simulink model "TorqueVect"  (R2022a)
settings: Solver=VariableStepAuto  StartTime=0.0  StopTime=32  RelTol=1e-3
PreLoadFcn:
  | run('Parameters\FSE_Parameters.m')
undefined symbols (not defined in the file): BRegenEnabledButton, canChannel, CyalphaLookUp, efficiency, Fz_curve, Fz_scaling_long, gearR, izz, jw, Kd, kd, Ki, ki, Kp, kp, l_f, l_r, lambda, m, Mz_max, N, N_lat, N_long, P_max, pid_kd_lat, pid_kd_long, pid_ki_lat, pid_ki_long, pid_kp_lat, pid_kp_long, R_max, rw, steerR, T_i_max, TC_Decr_Gas, TC_Derivative, TC_Incr_Gas, TC_On, TC_Relay_Off, TC_Relay_On, tireCornerStiffness, Ts, TV_On, TV_Override, velocity_lookup, velocity_lookup_lat, y_ref, yrr_scaling
libraries: simulink x218, slpidlib x135, CarMaker4SL x101, TractionControlLibrary x13, canmsglib x9, canlib x8, TorqueVectoringLibrary x6, simulink_extras x4, PedalConversionLibrary x3, PowerControlLibrary x1
(part 6 of 26)

== system TorqueVect/CarMaker/IPG Vehicle/PowerTrain/PTControl Example/PTControl_PC_MFE/New TC ==
  lim 1 : Inport
  lim 2 : Inport  Port=2
  lim 3 : Inport  Port=3
  lim 4 : Inport  Port=4
  vx : Inport  Port=5
  w_FL : Inport  Port=6
  w_FR : Inport  Port=7
  w_RL : Inport  Port=8
  w_RR : Inport  Port=9
  Front SR Target : Inport  Port=10
  Rear SR Target : Inport  Port=11
  P_TC : Inport  Port=12
  D_TC : Inport  Port=13
  enable_tc : Inport  Port=14
  rate_h : Inport  Port=15
  rate_l : Inport  Port=16
  Demux1 : Demux
  Gain : Gain  Gain=0.2032/13.39
  Rate Limiter Dynamic{,1..3} (4 alike) : simulink/Discontinuities/Rate Limiter Dynamic
  Reference Generator1 : Subsystem
  Saturation : Saturate  UpperLimit=inf  LowerLimit=0
  Subtract1 : Sum  Inputs=-+
  TC R1 : Subsystem
  TC R2 : Subsystem
  TC R3 : Subsystem
  TC R4 : Subsystem
  Vector Concatenate3 : Concatenate  NumInputs=4
  R1 Demand : Outport
  L1 Demand : Outport  Port=2
  R2 Demand : Outport  Port=3
  L2 Demand : Outport  Port=4
  wires:
  Reference Generator1/1(R1) -> TC R1/1(modified slip ratio reference)
  lim 1/1 -> TC R1/2(lim 1)
  Gain/1 -> Subtract1/2
  Vector Concatenate3/1 -> Gain/1  "omega"
  Subtract1/1 -> Demux1/1
  vx/1 -> Saturation/1
  TC R2/1(Control Effort 1) -> Rate Limiter Dynamic1/2  "MMotorL1Demand"
  w_RL/1 -> Vector Concatenate3/4
  w_RR/1 -> Vector Concatenate3/3
  w_FL/1 -> Vector Concatenate3/2
  w_FR/1 -> Vector Concatenate3/1
  Front SR Target/1 -> Reference Generator1/2(Front SR Target)
  Rear SR Target/1 -> Reference Generator1/3(Rear SR Target)
  lim 2/1 -> TC R2/2(lim 1)
  lim 3/1 -> TC R3/2(lim 1)
  lim 4/1 -> TC R4/2(lim 1)
  Reference Generator1/2(L1) -> TC R2/1(modified slip ratio reference)
  Reference Generator1/3(R2) -> TC R3/1(modified slip ratio reference)
  Reference Generator1/4(L2) -> TC R4/1(modified slip ratio reference)
  P_TC/1 -> TC R2/4(P_TC), TC R4/4(P_TC), TC R3/4(P_TC), TC R1/4(P_TC)
  D_TC/1 -> TC R2/5(D_TC), TC R4/5(D_TC), TC R3/5(D_TC), TC R1/5(D_TC)
  Demux1/1 -> TC R1/3(modified slip ratio measurement)
  Demux1/2 -> TC R2/3(modified slip ratio measurement)
  Demux1/3 -> TC R3/3(modified slip ratio measurement)
  Demux1/4 -> TC R4/3(modified slip ratio measurement)
  TC R1/1(Control Effort 1) -> Rate Limiter Dynamic/2  "MMotorR1Demand"
  Saturation/1 -> Subtract1/1, Reference Generator1/1(x2)
  TC R3/1(Control Effort 1) -> Rate Limiter Dynamic2/2
  TC R4/1(Control Effort 1) -> Rate Limiter Dynamic3/2
  enable_tc/1 -> TC R4/6(enable_tc), TC R2/6(enable_tc), TC R3/6(enable_tc), TC R1/6(enable_tc)
  Rate Limiter Dynamic/1 -> R1 Demand/1
  rate_h/1 -> Rate Limiter Dynamic3/1, Rate Limiter Dynamic2/1, Rate Limiter Dynamic1/1, Rate Limiter Dynamic/1
  rate_l/1 -> Rate Limiter Dynamic/3, Rate Limiter Dynamic3/3, Rate Limiter Dynamic2/3, Rate Limiter Dynamic1/3
  Rate Limiter Dynamic1/1 -> L1 Demand/1
  Rate Limiter Dynamic2/1 -> R2 Demand/1
  Rate Limiter Dynamic3/1 -> L2 Demand/1

== system TorqueVect/CarMaker/IPG Vehicle/PowerTrain/PTControl Example/PTControl_PC_MFE/PTC ==
  Constant2 : Constant
  Ground : Ground
  Mode_EngineDrive : Constant  Value=4
  Mux : Mux
  OperState_Driving : Constant  Value=4
  PTC MiscOut : Outport  VectorParamsAs1DForOutWhenUnconnected=off
  wires:
  Constant2/1 -> Mux/4  "Ignition"
  Mode_EngineDrive/1 -> Mux/3
  Ground/1 -> Mux/2  "OperationError"
  OperState_Driving/1 -> Mux/1
  Mux/1 -> PTC MiscOut/1

== system TorqueVect/CarMaker/IPG Vehicle/PowerTrain/PTControl Example/PTControl_PC_MFE/Subsystem ==
  rThrottlePedal : Inport
  vLong : Inport  Port=2
  BRegenEnabledButton : Inport  Port=3
  MMotorFL : Inport  Port=4
  MMotorFR : Inport  Port=5
  MMotorRL : Inport  Port=6
  MMotorRR : Inport  Port=7
  nMotorFL : Inport  Port=8
  nMotorFR : Inport  Port=9
  nMotorRL : Inport  Port=10
  nMotorRR : Inport  Port=11
  PMeasured : Inport  Port=12
  BMeasuredEnable : Inport  Port=13
  rSplitF : Inport  Port=14
  rRegenSplitF : Inport  Port=15
  PRegenLimit : Inport  Port=16
  PLimit : Inport  Port=17
  FF_PC : Inport  Port=18
  FF_RC : Inport  Port=19
  P_PC : Inport  Port=20
  D_PC : Inport  Port=21
  MMotorMax : Inport  Port=22
  Add{,1..3} (4 alike) : Sum  Inputs=-+
  PedalConversion : PedalConversionLibrary/PedalConversion  SystemSampleTime=-1  VariantActivationTime=update diagram  Latency=0  AutoFrameSizeCalculation=off
  PowerControl : Subsystem  AncestorBlock=PowerControlLibrary/PowerControl
  TorqueSplit : TorqueVectoringLibrary/TorqueSplit  SystemSampleTime=-1  VariantActivationTime=update diagram  Latency=0  AutoFrameSizeCalculation=off
  MMotorDemandFL : Outport
  MMotorDemandFR : Outport  Port=2
  MMotorDemandRL : Outport  Port=3
  MMotorDemandRR : Outport  Port=4
  wires:
  rThrottlePedal/1 -> [rThrottlePedal]
  [rThrottlePedal] -> PedalConversion/1
  [rThrottlePedal] -> PowerControl/13(rThrottlePedal)
  vLong/1 -> PedalConversion/3
  BRegenEnabledButton/1 -> PedalConversion/2
  MMotorFL/1 -> PowerControl/1(MMotorFL)
  MMotorFR/1 -> PowerControl/2(MMotorFR)
  MMotorRL/1 -> PowerControl/3(MMotorRL)
  MMotorRR/1 -> PowerControl/4(MMotorRR)
  nMotorFL/1 -> PowerControl/5(nMotorFL)
  nMotorFR/1 -> PowerControl/6(nMotorFR)
  nMotorRL/1 -> PowerControl/7(nMotorRL)
  nMotorRR/1 -> PowerControl/8(nMotorRR)
  PMeasured/1 -> PowerControl/9(PMeasured)
  BMeasuredEnable/1 -> PowerControl/10(BMeasuredEnable)
  PRegenLimit/1 -> PowerControl/15(PRegenLimit)
  PLimit/1 -> PowerControl/16(PLimit)
  FF_PC/1 -> PowerControl/17(FF_PC)
  FF_RC/1 -> PowerControl/18(FF_RC)
  P_PC/1 -> PowerControl/19(P_PC)
  D_PC/1 -> PowerControl/20(D_PC)
  Add/1 -> MMotorDemandFL/1
  PowerControl/1(MReductionMotorFL) -> Add/1
  rSplitF/1 -> [rSplitF]
  [rSplitF] -> TorqueSplit/1
  rRegenSplitF/1 -> TorqueSplit/2
  PedalConversion/1 -> PowerControl/14(rThrottle), TorqueSplit/3
  MMotorMax/1 -> TorqueSplit/4
  [rSplitF] -> PowerControl/12(rSplitF)
  PedalConversion/2 -> PowerControl/11(BRegenEnable)
  TorqueSplit/1 -> [MMotorRequestFL]
  TorqueSplit/2 -> [MMotorRequestFR]
  TorqueSplit/3 -> [MMotorRequestRL]
  TorqueSplit/4 -> [MMotorRequestRR]
  [MMotorRequestFL] -> Add/2
  Add1/1 -> MMotorDemandFR/1
  PowerControl/2(MReductionMotorFR) -> Add1/1
  [MMotorRequestFR] -> Add1/2
  Add2/1 -> MMotorDemandRL/1
  PowerControl/3(MReductionMotorRL) -> Add2/1
  [MMotorRequestRL] -> Add2/2
  Add3/1 -> MMotorDemandRR/1
  PowerControl/4(MReductionMotorRR) -> Add3/1
  [MMotorRequestRR] -> Add3/2

== system TorqueVect/CarMaker/IPG Vehicle/PowerTrain/PTControl Example/PTControl_PC_TC_MFE/New TC ==
  lim 1 : Inport
  lim 2 : Inport  Port=2
  lim 3 : Inport  Port=3
  lim 4 : Inport  Port=4
  vx : Inport  Port=5
  w_FL : Inport  Port=6
  w_FR : Inport  Port=7
  w_RL : Inport  Port=8
  w_RR : Inport  Port=9
  Front SR Target : Inport  Port=10
  Rear SR Target : Inport  Port=11
  P_TC : Inport  Port=12
  D_TC : Inport  Port=13
  enable_tc : Inport  Port=14
  rate_h : Inport  Port=15
  rate_l : Inport  Port=16
  Demux1 : Demux
  Gain : Gain  Gain=0.2032/13.39
  Rate Limiter Dynamic{,1..3} (4 alike) : simulink/Discontinuities/Rate Limiter Dynamic
  Reference Generator1 : Subsystem
  Saturation : Saturate  UpperLimit=inf  LowerLimit=0
  Subtract1 : Sum  Inputs=-+
  TC R1 : Subsystem
  TC R2 : Subsystem
  TC R3 : Subsystem
  TC R4 : Subsystem
  Vector Concatenate3 : Concatenate  NumInputs=4
  R1 Demand : Outport
  L1 Demand : Outport  Port=2
  R2 Demand : Outport  Port=3
  L2 Demand : Outport  Port=4
  wires:
  Reference Generator1/1(R1) -> TC R1/1(modified slip ratio reference)
  lim 1/1 -> TC R1/2(lim 1)
  Gain/1 -> Subtract1/2
  Vector Concatenate3/1 -> Gain/1  "omega"
  Subtract1/1 -> Demux1/1
  vx/1 -> Saturation/1
  TC R2/1(Control Effort 1) -> Rate Limiter Dynamic1/2  "MMotorL1Demand"
  w_RL/1 -> Vector Concatenate3/4
  w_RR/1 -> Vector Concatenate3/3
  w_FL/1 -> Vector Concatenate3/2
  w_FR/1 -> Vector Concatenate3/1
  Front SR Target/1 -> Reference Generator1/2(Front SR Target)
  Rear SR Target/1 -> Reference Generator1/3(Rear SR Target)
  lim 2/1 -> TC R2/2(lim 1)
  lim 3/1 -> TC R3/2(lim 1)
  lim 4/1 -> TC R4/2(lim 1)
  Reference Generator1/2(L1) -> TC R2/1(modified slip ratio reference)
  Reference Generator1/3(R2) -> TC R3/1(modified slip ratio reference)
  Reference Generator1/4(L2) -> TC R4/1(modified slip ratio reference)
  P_TC/1 -> TC R2/4(P_TC), TC R4/4(P_TC), TC R3/4(P_TC), TC R1/4(P_TC)
  D_TC/1 -> TC R2/5(D_TC), TC R4/5(D_TC), TC R3/5(D_TC), TC R1/5(D_TC)
  Demux1/1 -> TC R1/3(modified slip ratio measurement)
  Demux1/2 -> TC R2/3(modified slip ratio measurement)
  Demux1/3 -> TC R3/3(modified slip ratio measurement)
  Demux1/4 -> TC R4/3(modified slip ratio measurement)
  TC R1/1(Control Effort 1) -> Rate Limiter Dynamic/2  "MMotorR1Demand"
  Saturation/1 -> Subtract1/1, Reference Generator1/1(x2)
  TC R3/1(Control Effort 1) -> Rate Limiter Dynamic2/2
  TC R4/1(Control Effort 1) -> Rate Limiter Dynamic3/2
  enable_tc/1 -> TC R4/6(enable_tc), TC R2/6(enable_tc), TC R3/6(enable_tc), TC R1/6(enable_tc)
  Rate Limiter Dynamic/1 -> R1 Demand/1
  rate_h/1 -> Rate Limiter Dynamic3/1, Rate Limiter Dynamic2/1, Rate Limiter Dynamic1/1, Rate Limiter Dynamic/1
  rate_l/1 -> Rate Limiter Dynamic/3, Rate Limiter Dynamic3/3, Rate Limiter Dynamic2/3, Rate Limiter Dynamic1/3
  Rate Limiter Dynamic1/1 -> L1 Demand/1
  Rate Limiter Dynamic2/1 -> R2 Demand/1
  Rate Limiter Dynamic3/1 -> L2 Demand/1

== system TorqueVect/CarMaker/IPG Vehicle/PowerTrain/PTControl Example/PTControl_PC_TC_MFE/PTC ==
  Constant2 : Constant
  Ground : Ground
  Mode_EngineDrive : Constant  Value=4
  Mux : Mux
  OperState_Driving : Constant  Value=4
  PTC MiscOut : Outport  VectorParamsAs1DForOutWhenUnconnected=off
  wires:
  Constant2/1 -> Mux/4  "Ignition"
  Mode_EngineDrive/1 -> Mux/3
  Ground/1 -> Mux/2  "OperationError"
  OperState_Driving/1 -> Mux/1
  Mux/1 -> PTC MiscOut/1

== system TorqueVect/CarMaker/IPG Vehicle/PowerTrain/PTControl Example/PTControl_PC_TC_MFE/Subsystem1 ==
  rThrottlePedal : Inport
  vLong : Inport  Port=2
  BRegenEnabledButton : Inport  Port=3
  MMotorFL : Inport  Port=4
  MMotorFR : Inport  Port=5
  MMotorRL : Inport  Port=6
  MMotorRR : Inport  Port=7
  rSlipTargetF : Inport  Port=8
  rSlipTargetR : Inport  Port=9
  BEnableTC : Inport  Port=10
  P_TC : Inport  Port=11
  PMeasured : Inport  Port=12
  D_TC : Inport  Port=13
  BMeasuredEnable : Inport  Port=14
  FF_TC : Inport  Port=15
  rSplitF : Inport  Port=16
  rLimitHigh : Inport  Port=17
  rRegenSplitF : Inport  Port=18
  PRegenLimit : Inport  Port=19
  rLimitLow : Inport  Port=20
  PLimit : Inport  Port=21
  FF_PC : Inport  Port=22
  FF_RC : Inport  Port=23
  P_PC : Inport  Port=24
  D_PC : Inport  Port=25
  MMotorMax : Inport  Port=26
  nMotorFL : Inport  Port=27
  nMotorFR : Inport  Port=28
  nMotorRL : Inport  Port=29
  nMotorRR : Inport  Port=30
  Subsystem : Subsystem
  TC : Subsystem
  MMotorDemandFL : Outport
  MMotorDemandFR : Outport  Port=2
  MMotorDemandRL : Outport  Port=3
  MMotorDemandRR : Outport  Port=4
  wires:
  [nMotorRL] -> Subsystem/10(nMotorRL)
  PRegenLimit/1 -> Subsystem/16(PRegenLimit)
  Subsystem/1(MMotorDemandFL) -> TC/14(MMotorRequestFL)
  [nMotorFL] -> Subsystem/8(nMotorFL)
  FF_TC/1 -> TC/11(FF_TC)
  Subsystem/3(MMotorDemandRL) -> TC/16(MMotorRequestRL)
  Subsystem/2(MMotorDemandFR) -> TC/15(MMotorRequestFR)
  rRegenSplitF/1 -> Subsystem/15(rRegenSplitF)
  BMeasuredEnable/1 -> Subsystem/13(BMeasuredEnable)
  MMotorMax/1 -> Subsystem/22(MMotorMax)
  Subsystem/4(MMotorDemandRR) -> TC/17(MMotorRequestRR)
  FF_PC/1 -> Subsystem/18(FF_PC)
  D_PC/1 -> Subsystem/21(D_PC)
  rLimitLow/1 -> TC/13(rLimitLow)
  TC/3(MMotorDemandRL) -> MMotorDemandRL/1
  [nMotorFR] -> Subsystem/9(nMotorFR)
  TC/4(MMotorDemandRR) -> MMotorDemandRR/1
  D_TC/1 -> TC/10(D_TC)
  PLimit/1 -> Subsystem/17(PLimit)
  P_PC/1 -> Subsystem/20(P_PC)
  FF_RC/1 -> Subsystem/19(FF_RC)
  vLong/1 -> TC/1(vLong), Subsystem/2(vLong)
  [nMotorFL] -> TC/2(nMotorFL)
  [nMotorRL] -> TC/4(nMotorRL)
  TC/1(MMotorDemandFL) -> MMotorDemandFL/1
  MMotorRL/1 -> Subsystem/6(MMotorRL)
  P_TC/1 -> TC/9(P_TC)
  MMotorFL/1 -> Subsystem/4(MMotorFL)
  [nMotorFR] -> TC/3(nMotorFR)
  [nMotorRR] -> TC/5(nMotorRR)
  rSlipTargetF/1 -> TC/6(rSlipTargetF)
  rSlipTargetR/1 -> TC/7(rSlipTargetR)
  rLimitHigh/1 -> TC/12(rLimitHigh)
  BEnableTC/1 -> TC/8(BEnableTC)
  BRegenEnabledButton/1 -> Subsystem/3(BRegenEnabledButton)
  rSplitF/1 -> Subsystem/14(rSplitF)
  [nMotorRR] -> Subsystem/11(nMotorRR)
  MMotorFR/1 -> Subsystem/5(MMotorFR)
  MMotorRR/1 -> Subsystem/7(MMotorRR)
  TC/2(MMotorDemandFR) -> MMotorDemandFR/1
  rThrottlePedal/1 -> Subsystem/1(rThrottlePedal)
  PMeasured/1 -> Subsystem/12(PMeasured)
  nMotorFL/1 -> [nMotorFL]
  nMotorFR/1 -> [nMotorFR]
  nMotorRL/1 -> [nMotorRL]
  nMotorRR/1 -> [nMotorRR]

== system TorqueVect/CarMaker/IPG Vehicle/PowerTrain/PTControl Example/PTControl_TC_MFE/New TC ==
  lim 1 : Inport
  lim 2 : Inport  Port=2
  lim 3 : Inport  Port=3
  lim 4 : Inport  Port=4
  vx : Inport  Port=5
  w_FL : Inport  Port=6
  w_FR : Inport  Port=7
  w_RL : Inport  Port=8
  w_RR : Inport  Port=9
  Front SR Target : Inport  Port=10
  Rear SR Target : Inport  Port=11
  P_TC : Inport  Port=12
  D_TC : Inport  Port=13
  enable_tc : Inport  Port=14
  rate_h : Inport  Port=15
  rate_l : Inport  Port=16
  Demux1 : Demux
  Gain : Gain  Gain=0.2032/13.39
  Rate Limiter Dynamic{,1..3} (4 alike) : simulink/Discontinuities/Rate Limiter Dynamic
  Reference Generator1 : Subsystem
  Saturation : Saturate  UpperLimit=inf  LowerLimit=0
  Subtract1 : Sum  Inputs=-+
  TC R1 : Subsystem
  TC R2 : Subsystem
  TC R3 : Subsystem
  TC R4 : Subsystem
  Vector Concatenate3 : Concatenate  NumInputs=4
  R1 Demand : Outport
  L1 Demand : Outport  Port=2
  R2 Demand : Outport  Port=3
  L2 Demand : Outport  Port=4
  wires:
  Reference Generator1/1(R1) -> TC R1/1(modified slip ratio reference)
  lim 1/1 -> TC R1/2(lim 1)
  Gain/1 -> Subtract1/2
  Vector Concatenate3/1 -> Gain/1  "omega"
  Subtract1/1 -> Demux1/1
  vx/1 -> Saturation/1
  TC R2/1(Control Effort 1) -> Rate Limiter Dynamic1/2  "MMotorL1Demand"
  w_RL/1 -> Vector Concatenate3/4
  w_RR/1 -> Vector Concatenate3/3
  w_FL/1 -> Vector Concatenate3/2
  w_FR/1 -> Vector Concatenate3/1
  Front SR Target/1 -> Reference Generator1/2(Front SR Target)
  Rear SR Target/1 -> Reference Generator1/3(Rear SR Target)
  lim 2/1 -> TC R2/2(lim 1)
  lim 3/1 -> TC R3/2(lim 1)
  lim 4/1 -> TC R4/2(lim 1)
  Reference Generator1/2(L1) -> TC R2/1(modified slip ratio reference)
  Reference Generator1/3(R2) -> TC R3/1(modified slip ratio reference)
  Reference Generator1/4(L2) -> TC R4/1(modified slip ratio reference)
  P_TC/1 -> TC R2/4(P_TC), TC R4/4(P_TC), TC R3/4(P_TC), TC R1/4(P_TC)
  D_TC/1 -> TC R2/5(D_TC), TC R4/5(D_TC), TC R3/5(D_TC), TC R1/5(D_TC)
  Demux1/1 -> TC R1/3(modified slip ratio measurement)
  Demux1/2 -> TC R2/3(modified slip ratio measurement)
  Demux1/3 -> TC R3/3(modified slip ratio measurement)
  Demux1/4 -> TC R4/3(modified slip ratio measurement)
  TC R1/1(Control Effort 1) -> Rate Limiter Dynamic/2  "MMotorR1Demand"
  Saturation/1 -> Subtract1/1, Reference Generator1/1(x2)
  TC R3/1(Control Effort 1) -> Rate Limiter Dynamic2/2
  TC R4/1(Control Effort 1) -> Rate Limiter Dynamic3/2
  enable_tc/1 -> TC R4/6(enable_tc), TC R2/6(enable_tc), TC R3/6(enable_tc), TC R1/6(enable_tc)
  Rate Limiter Dynamic/1 -> R1 Demand/1
  rate_h/1 -> Rate Limiter Dynamic3/1, Rate Limiter Dynamic2/1, Rate Limiter Dynamic1/1, Rate Limiter Dynamic/1
  rate_l/1 -> Rate Limiter Dynamic/3, Rate Limiter Dynamic3/3, Rate Limiter Dynamic2/3, Rate Limiter Dynamic1/3
  Rate Limiter Dynamic1/1 -> L1 Demand/1
  Rate Limiter Dynamic2/1 -> R2 Demand/1
  Rate Limiter Dynamic3/1 -> L2 Demand/1

== system TorqueVect/CarMaker/IPG Vehicle/PowerTrain/PTControl Example/PTControl_TC_MFE/PTC ==
  Constant2 : Constant
  Ground : Ground
  Mode_EngineDrive : Constant  Value=4
  Mux : Mux
  OperState_Driving : Constant  Value=4
  PTC MiscOut : Outport  VectorParamsAs1DForOutWhenUnconnected=off
  wires:
  Constant2/1 -> Mux/4  "Ignition"
  Mode_EngineDrive/1 -> Mux/3
  Ground/1 -> Mux/2  "OperationError"
  OperState_Driving/1 -> Mux/1
  Mux/1 -> PTC MiscOut/1

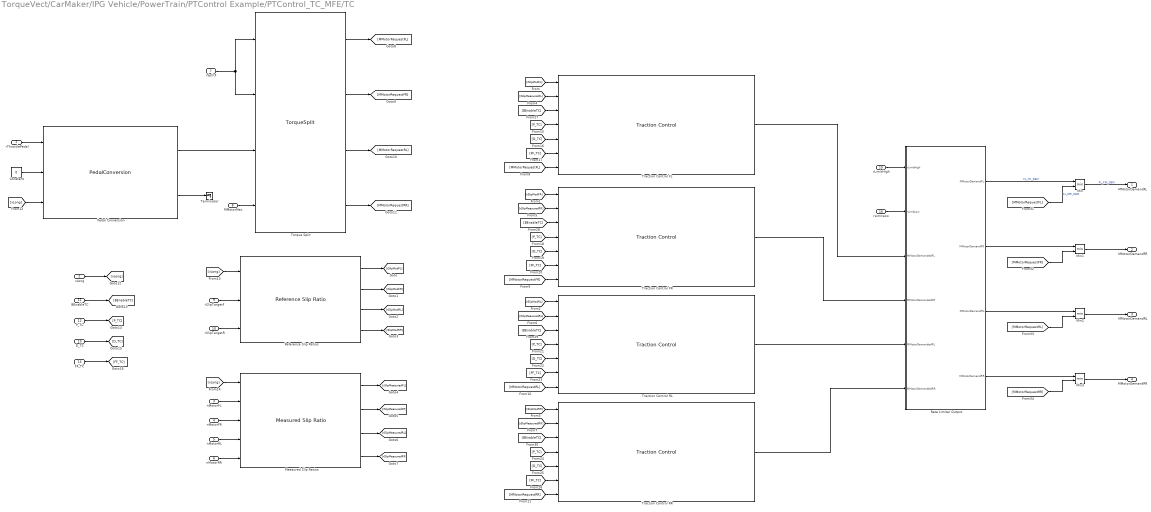
== system TorqueVect/CarMaker/IPG Vehicle/PowerTrain/PTControl Example/PTControl_TC_MFE/TC ==
  rThrottlePedal : Inport
  vLong : Inport  Port=2
  nMotorFL : Inport  Port=3
  nMotorFR : Inport  Port=4
  nMotorRL : Inport  Port=5
  nMotorRR : Inport  Port=6
  rSplitF : Inport  Port=7
  MMotorMax : Inport  Port=8
  rSlipTargetF : Inport  Port=9
  rSlipTargetR : Inport  Port=10
  BEnableTC : Inport  Port=11
  P_TC : Inport  Port=12
  D_TC : Inport  Port=13
  FF_TC : Inport  Port=14
  rLimitHigh : Inport  Port=15
  rLimitLow : Inport  Port=16
  Constant : Constant  Value=0
  Measured Slip Ratios : TractionControlLibrary/Measured Slip Ratio  SystemSampleTime=-1  VariantActivationTime=update diagram  Latency=0  AutoFrameSizeCalculation=off
  Min{,1..3} (4 alike) : MinMax  Inputs=2
  Pedal Conversion : PedalConversionLibrary/PedalConversion  SystemSampleTime=-1  VariantActivationTime=update diagram  Latency=0  AutoFrameSizeCalculation=off
  Rate Limiter Output : Subsystem  AncestorBlock=TractionControlLibrary/Rate Limiter
  Reference Slip Ratios : TractionControlLibrary/Reference Slip Ratio  SystemSampleTime=-1  VariantActivationTime=update diagram  Latency=0  AutoFrameSizeCalculation=off
  Terminator : Terminator
  Torque Split : TorqueVectoringLibrary/TorqueSplit  SystemSampleTime=-1  VariantActivationTime=update diagram  Latency=0  AutoFrameSizeCalculation=off
  Traction Control FL : TractionControlLibrary/Traction Control  SystemSampleTime=-1  VariantActivationTime=update diagram  Latency=0  AutoFrameSizeCalculation=off
  Traction Control FR : TractionControlLibrary/Traction Control  SystemSampleTime=-1  VariantActivationTime=update diagram  Latency=0  AutoFrameSizeCalculation=off
  Traction Control RL : TractionControlLibrary/Traction Control  SystemSampleTime=-1  VariantActivationTime=update diagram  Latency=0  AutoFrameSizeCalculation=off
  Traction Control RR : TractionControlLibrary/Traction Control  SystemSampleTime=-1  VariantActivationTime=update diagram  Latency=0  AutoFrameSizeCalculation=off
  MMotorDemandFL : Outport
  MMotorDemandFR : Outport  Port=2
  MMotorDemandRL : Outport  Port=3
  MMotorDemandRR : Outport  Port=4
  wires:
  Traction Control FL/1 -> Rate Limiter Output/3(MMotorDemandedFL)
  Traction Control FR/1 -> Rate Limiter Output/4(MMotorDemandedFR)
  Traction Control RL/1 -> Rate Limiter Output/5(MMotorDemandedRL)
  Traction Control RR/1 -> Rate Limiter Output/6(MMotorDemandedRR)
  Reference Slip Ratios/1 -> [rSlipModFL]
  Reference Slip Ratios/2 -> [rSlipModFR]
  Reference Slip Ratios/3 -> [rSlipModRL]
  Reference Slip Ratios/4 -> [rSlipModRR]
  [rSlipModFL] -> Traction Control FL/1
  [rSlipModFR] -> Traction Control FR/1
  [rSlipModRL] -> Traction Control RL/1
  [rSlipModRR] -> Traction Control RR/1
  Measured Slip Ratios/1 -> [rSlipMeasuredFL]
  Measured Slip Ratios/2 -> [rSlipMeasuredFR]
  Measured Slip Ratios/3 -> [rSlipMeasuredRL]
  Measured Slip Ratios/4 -> [rSlipMeasuredRR]
  [rSlipMeasuredFL] -> Traction Control FL/2
  [rSlipMeasuredFR] -> Traction Control FR/2
  [rSlipMeasuredRL] -> Traction Control RL/2
  [rSlipMeasuredRR] -> Traction Control RR/2
  Torque Split/1 -> [MMotorRequestFL]
  Torque Split/2 -> [MMotorRequestFR]
  Torque Split/3 -> [MMotorRequestRL]
  Torque Split/4 -> [MMotorRequestRR]
  [MMotorRequestFL] -> Traction Control FL/7
  [MMotorRequestFR] -> Traction Control FR/7
  [MMotorRequestRL] -> Traction Control RL/7
  [MMotorRequestRR] -> Traction Control RR/7
  Pedal Conversion/1 -> Torque Split/3
  Pedal Conversion/2 -> Terminator/1
  Constant/1 -> Pedal Conversion/2
  rThrottlePedal/1 -> Pedal Conversion/1
  vLong/1 -> [vLong]
  [vLong] -> Pedal Conversion/3
  [vLong] -> Reference Slip Ratios/1
  [vLong] -> Measured Slip Ratios/1
  nMotorFL/1 -> Measured Slip Ratios/2
  nMotorFR/1 -> Measured Slip Ratios/3
  nMotorRL/1 -> Measured Slip Ratios/4
  nMotorRR/1 -> Measured Slip Ratios/5
  rSplitF/1 -> Torque Split/2, Torque Split/1
  MMotorMax/1 -> Torque Split/4
  rSlipTargetF/1 -> Reference Slip Ratios/2
  rSlipTargetR/1 -> Reference Slip Ratios/3
  BEnableTC/1 -> [BEnableTC]
  P_TC/1 -> [P_TC]
  D_TC/1 -> [D_TC]
  FF_TC/1 -> [FF_TC]
  [P_TC] -> Traction Control FL/4
  [D_TC] -> Traction Control FL/5
  [FF_TC] -> Traction Control FL/6
  [FF_TC] -> Traction Control FR/6
  [D_TC] -> Traction Control FR/5
  [P_TC] -> Traction Control FR/4
  [FF_TC] -> Traction Control RL/6
  [D_TC] -> Traction Control RL/5
  [P_TC] -> Traction Control RL/4
  [FF_TC] -> Traction Control RR/6
  [D_TC] -> Traction Control RR/5
  [P_TC] -> Traction Control RR/4
  [BEnableTC] -> Traction Control FL/3
  [BEnableTC] -> Traction Control FR/3
  [BEnableTC] -> Traction Control RL/3
  [BEnableTC] -> Traction Control RR/3
  rLimitHigh/1 -> Rate Limiter Output/1(rLimitHigh)
  rLimitLow/1 -> Rate Limiter Output/2(rLimitLow)
  Rate Limiter Output/1(MMotorDemandFL) -> Min/1  "FL_TC_DEM"
  [MMotorRequestFL] -> Min/2  "FL_ORI_DEM"
  Min/1 -> MMotorDemandFL/1  "FL_FIN_DEM"
  Rate Limiter Output/2(MMotorDemandFR) -> Min1/1
  Min1/1 -> MMotorDemandFR/1
  [MMotorRequestFR] -> Min1/2
  Rate Limiter Output/3(MMotorDemandRL) -> Min2/1
  Min2/1 -> MMotorDemandRL/1
  [MMotorRequestRL] -> Min2/2
  Rate Limiter Output/4(MMotorDemandRR) -> Min3/1
  Min3/1 -> MMotorDemandRR/1
  [MMotorRequestRR] -> Min3/2

== system TorqueVect/CarMaker/IPG Vehicle/PowerTrain/PTControl Example/PTControl_TV_IPG/PTC ==
  Constant2 : Constant
  Ground : Ground
  Mode_EngineDrive : Constant  Value=4
  Mux : Mux
  OperState_Driving : Constant  Value=4
  PTC MiscOut : Outport  VectorParamsAs1DForOutWhenUnconnected=off
  wires:
  Constant2/1 -> Mux/4  "Ignition"
  Mode_EngineDrive/1 -> Mux/3
  Ground/1 -> Mux/2  "OperationError"
  OperState_Driving/1 -> Mux/1
  Mux/1 -> PTC MiscOut/1

== system TorqueVect/CarMaker/IPG Vehicle/PowerTrain/PTControl Example/PTControl_TV_IPG/Torque Control 0 ==
  note: Load_Motor0_FL
  note: Trq_trg
  Gas : Inport
  Add : Sum
  Constant2 : Constant  Value=TC_On
  Constant4 : Constant  Value=TV_On
  Electronic Gas Pedal FL : Subsystem
  Mux : Mux  Inputs=3
  NOTSET1 : Constant  Value=-99999
  NOTSET3 : Constant  Value=-99999
  Product1 : Product  RndMeth=Zero
  Scope : Scope
  Torque Vectoring FL : Subsystem
  MotorOut0 : Outport  VectorParamsAs1DForOutWhenUnconnected=off
  wires:
  Gas/1 -> Electronic Gas Pedal FL/2(VC.Gas)
  NOTSET1/1 -> Mux/3  "rotv_trg"
  NOTSET3/1 -> Mux/2
  Add/1 -> Scope/1, Mux/1
  Product1/1 -> Add/2
  Constant4/1 -> Product1/2
  Torque Vectoring FL/1(TV FL) -> Product1/1
  Electronic Gas Pedal FL/1(Motor_Gas_FL) -> Add/1
  Constant2/1 -> Electronic Gas Pedal FL/1(TV_On)
  Mux/1 -> MotorOut0/1

== system TorqueVect/CarMaker/IPG Vehicle/PowerTrain/PTControl Example/PTControl_TV_IPG/Torque Control 1 ==
  note: Trq_trg
  note: Load_Motor1_FR
  Gas : Inport
  Add : Sum
  Constant2 : Constant  Value=TC_On
  Constant4 : Constant  Value=TV_On
  Electronic Gas Pedal FR : Subsystem
  Mux : Mux  Inputs=3
  NOTSET1 : Constant  Value=-99999
  NOTSET3 : Constant  Value=-99999
  Product1 : Product  RndMeth=Zero
  Torque Vectoring FR : Subsystem
  MotorOut1 : Outport  VectorParamsAs1DForOutWhenUnconnected=off
  wires:
  Gas/1 -> Electronic Gas Pedal FR/2(VC.Gas)
  Mux/1 -> MotorOut1/1
  Constant2/1 -> Electronic Gas Pedal FR/1(TV_On)
  Electronic Gas Pedal FR/1(Motor_Gas_FR) -> Add/1
  Torque Vectoring FR/1(TV FR) -> Product1/1
  Constant4/1 -> Product1/2
  Product1/1 -> Add/2
  Add/1 -> Mux/1
  NOTSET3/1 -> Mux/2
  NOTSET1/1 -> Mux/3  "rotv_trg"

== system TorqueVect/CarMaker/IPG Vehicle/PowerTrain/PTControl Example/PTControl_TV_IPG/Torque Control 2 ==
  note: Trq_trg
  note: Load_Motor2_RL
  Gas : Inport
  Add : Sum
  Constant2 : Constant  Value=TC_On
  Constant4 : Constant  Value=TV_On
  Electronic Gas Pedal RL : Subsystem
  Mux : Mux  Inputs=3
  NOTSET1 : Constant  Value=-99999
  NOTSET3 : Constant  Value=-99999
  Product1 : Product  RndMeth=Zero
  Torque Vectoring RL : Subsystem
  MotorOut2 : Outport  VectorParamsAs1DForOutWhenUnconnected=off
  wires:
  Gas/1 -> Electronic Gas Pedal RL/2(VC.Gas)
  Mux/1 -> MotorOut2/1
  Constant2/1 -> Electronic Gas Pedal RL/1(TV_On)
  Electronic Gas Pedal RL/1(Motor_Gas_RL) -> Add/1
  Torque Vectoring RL/1(TV RL) -> Product1/1
  Constant4/1 -> Product1/2
  Product1/1 -> Add/2
  Add/1 -> Mux/1
  NOTSET3/1 -> Mux/2
  NOTSET1/1 -> Mux/3  "rotv_trg"

== system TorqueVect/CarMaker/IPG Vehicle/PowerTrain/PTControl Example/PTControl_TV_IPG/Torque Control 3 ==
  note: Load_Motor3_RR
  note: Trq_trg
  Gas : Inport
  Add : Sum
  Constant2 : Constant  Value=TC_On
  Constant4 : Constant  Value=TV_On
  Electronic Gas Pedal RR : Subsystem
  Mux : Mux  Inputs=3
  NOTSET1 : Constant  Value=-99999
  NOTSET3 : Constant  Value=-99999
  Product1 : Product  RndMeth=Zero
  Torque Vectoring RR : Subsystem
  MotorOut3 : Outport  VectorParamsAs1DForOutWhenUnconnected=off
  wires:
  Gas/1 -> Electronic Gas Pedal RR/2(VC.Gas)
  NOTSET1/1 -> Mux/3  "rotv_trg"
  NOTSET3/1 -> Mux/2
  Add/1 -> Mux/1
  Product1/1 -> Add/2
  Constant4/1 -> Product1/2
  Torque Vectoring RR/1(TV RR) -> Product1/1
  Electronic Gas Pedal RR/1(Motor_Gas_RR) -> Add/1
  Constant2/1 -> Electronic Gas Pedal RR/1(TV_On)
  Mux/1 -> MotorOut3/1

== system TorqueVect/CarMaker/IPG Vehicle/PowerTrain/PTControl Example/PTControl_TV_MFE1/New TC ==
  lim 1 : Inport
  lim 2 : Inport  Port=2
  lim 3 : Inport  Port=3
  lim 4 : Inport  Port=4
  vx : Inport  Port=5
  w_FL : Inport  Port=6
  w_FR : Inport  Port=7
  w_RL : Inport  Port=8
  w_RR : Inport  Port=9
  Front SR Target : Inport  Port=10
  Rear SR Target : Inport  Port=11
  P_TC : Inport  Port=12
  D_TC : Inport  Port=13
  enable_tc : Inport  Port=14
  rate_h : Inport  Port=15
  rate_l : Inport  Port=16
  Demux1 : Demux
  Gain : Gain  Gain=0.2032/13.39
  Rate Limiter Dynamic{,1..3} (4 alike) : simulink/Discontinuities/Rate Limiter Dynamic
  Reference Generator1 : Subsystem
  Saturation : Saturate  UpperLimit=inf  LowerLimit=0
  Subtract1 : Sum  Inputs=-+
  TC R1 : Subsystem
  TC R2 : Subsystem
  TC R3 : Subsystem
  TC R4 : Subsystem
  Vector Concatenate3 : Concatenate  NumInputs=4
  R1 Demand : Outport
  L1 Demand : Outport  Port=2
  R2 Demand : Outport  Port=3
  L2 Demand : Outport  Port=4
  wires:
  Reference Generator1/1(R1) -> TC R1/1(modified slip ratio reference)
  lim 1/1 -> TC R1/2(lim 1)
  Gain/1 -> Subtract1/2
  Vector Concatenate3/1 -> Gain/1  "omega"
  Subtract1/1 -> Demux1/1
  vx/1 -> Saturation/1
  TC R2/1(Control Effort 1) -> Rate Limiter Dynamic1/2  "MMotorL1Demand"
  w_RL/1 -> Vector Concatenate3/4
  w_RR/1 -> Vector Concatenate3/3
  w_FL/1 -> Vector Concatenate3/2
  w_FR/1 -> Vector Concatenate3/1
  Front SR Target/1 -> Reference Generator1/2(Front SR Target)
  Rear SR Target/1 -> Reference Generator1/3(Rear SR Target)
  lim 2/1 -> TC R2/2(lim 1)
  lim 3/1 -> TC R3/2(lim 1)
  lim 4/1 -> TC R4/2(lim 1)
  Reference Generator1/2(L1) -> TC R2/1(modified slip ratio reference)
  Reference Generator1/3(R2) -> TC R3/1(modified slip ratio reference)
  Reference Generator1/4(L2) -> TC R4/1(modified slip ratio reference)
  P_TC/1 -> TC R2/4(P_TC), TC R4/4(P_TC), TC R3/4(P_TC), TC R1/4(P_TC)
  D_TC/1 -> TC R2/5(D_TC), TC R4/5(D_TC), TC R3/5(D_TC), TC R1/5(D_TC)
  Demux1/1 -> TC R1/3(modified slip ratio measurement)
  Demux1/2 -> TC R2/3(modified slip ratio measurement)
  Demux1/3 -> TC R3/3(modified slip ratio measurement)
  Demux1/4 -> TC R4/3(modified slip ratio measurement)
  TC R1/1(Control Effort 1) -> Rate Limiter Dynamic/2  "MMotorR1Demand"
  Saturation/1 -> Subtract1/1, Reference Generator1/1(x2)
  TC R3/1(Control Effort 1) -> Rate Limiter Dynamic2/2
  TC R4/1(Control Effort 1) -> Rate Limiter Dynamic3/2
  enable_tc/1 -> TC R4/6(enable_tc), TC R2/6(enable_tc), TC R3/6(enable_tc), TC R1/6(enable_tc)
  Rate Limiter Dynamic/1 -> R1 Demand/1
  rate_h/1 -> Rate Limiter Dynamic3/1, Rate Limiter Dynamic2/1, Rate Limiter Dynamic1/1, Rate Limiter Dynamic/1
  rate_l/1 -> Rate Limiter Dynamic/3, Rate Limiter Dynamic3/3, Rate Limiter Dynamic2/3, Rate Limiter Dynamic1/3
  Rate Limiter Dynamic1/1 -> L1 Demand/1
  Rate Limiter Dynamic2/1 -> R2 Demand/1
  Rate Limiter Dynamic3/1 -> L2 Demand/1

== system TorqueVect/CarMaker/IPG Vehicle/PowerTrain/PTControl Example/PTControl_TV_MFE1/PTC ==
  Constant2 : Constant
  Ground : Ground
  Mode_EngineDrive : Constant  Value=4
  Mux : Mux
  OperState_Driving : Constant  Value=4
  PTC MiscOut : Outport  VectorParamsAs1DForOutWhenUnconnected=off
  wires:
  Constant2/1 -> Mux/4  "Ignition"
  Mode_EngineDrive/1 -> Mux/3
  Ground/1 -> Mux/2  "OperationError"
  OperState_Driving/1 -> Mux/1
  Mux/1 -> PTC MiscOut/1

== system TorqueVect/CarMaker/IPG Vehicle/PowerTrain/PTControl Example/PTControl_TV_MFE1/Subsystem ==
  vLong : Inport
  aSteerWheel : Inport  Port=2
  vLongMin : Inport  Port=3
  aSteerWheelMin : Inport  Port=4
  NTorqueMaxDeltaF : Inport  Port=5
  BTorqueVectoringEnable : Inport  Port=6
  rSplitF : Inport  Port=7
  P_YR : Inport  Port=8
  D_YR : Inport  Port=9
  rRegenSplitF : Inport  Port=10
  NBrake : Inport  Port=11
  rThrottle : Inport  Port=12
  MMotorMax : Inport  Port=13
  vLat : Inport  Port=14
  rSteerWheel : Inport  Port=15
  NTorqueMaxDeltaR : Inport  Port=16
  Add : Sum
  Add1 : Sum
  Enable : TorqueVectoringLibrary/Enable  SystemSampleTime=-1  VariantActivationTime=update diagram  Latency=0  AutoFrameSizeCalculation=off
  TorqueSplit : TorqueVectoringLibrary/TorqueSplit  SystemSampleTime=-1  VariantActivationTime=update diagram  Latency=0  AutoFrameSizeCalculation=off
  TorqueVectoringAlgorithm : Subsystem  AncestorBlock=TorqueVectoringLibrary/TorqueVectoringAlgorithm
  TorqueVectoringAlgorithm1 : Subsystem  AncestorBlock=TorqueVectoringLibrary/TorqueVectoringAlgorithm
  Vehicle Slip Angle Error : TorqueVectoringLibrary/Vehicle Slip Angle Error  SystemSampleTime=-1  VariantActivationTime=update diagram  Latency=0  AutoFrameSizeCalculation=off
  NTorqueLeftOut : Outport
  NTorqueRightOut : Outport  Port=2
  NTorqueLeftOut1 : Outport  Port=3
  NTorqueRightOut1 : Outport  Port=4
  wires:
  Vehicle Slip Angle Error/1 -> TorqueVectoringAlgorithm/5(aSlip), TorqueVectoringAlgorithm1/5(aSlip)
  TorqueSplit/4 -> Add1/2
  BTorqueVectoringEnable/1 -> Enable/5
  TorqueSplit/2 -> Add/2
  Enable/1 -> TorqueVectoringAlgorithm1/1(BEnable), TorqueVectoringAlgorithm/1(BEnable)  "Enable"
  rSteerWheel/1 -> Vehicle Slip Angle Error/4
  Add1/1 -> TorqueVectoringAlgorithm1/4(NTorqueAxle)
  TorqueVectoringAlgorithm1/2(NTorqueRightOut) -> NTorqueRightOut1/1
  NBrake/1 -> TorqueVectoringAlgorithm/8(NBrake), TorqueVectoringAlgorithm1/8(NBrake)
  rSplitF/1 -> TorqueSplit/1
  Add/1 -> TorqueVectoringAlgorithm/4(NTorqueAxle)
  TorqueSplit/3 -> Add1/1
  rThrottle/1 -> TorqueSplit/3
  vLong/1 -> Enable/1, Vehicle Slip Angle Error/2
  TorqueSplit/1 -> Add/1
  aSteerWheel/1 -> Vehicle Slip Angle Error/3, Enable/2
  vLongMin/1 -> Enable/3
  aSteerWheelMin/1 -> Enable/4
  D_YR/1 -> TorqueVectoringAlgorithm/7(D_YR), TorqueVectoringAlgorithm1/7(D_YR)
  MMotorMax/1 -> TorqueVectoringAlgorithm/3(NTorqueMax), TorqueVectoringAlgorithm1/3(NTorqueMax), TorqueSplit/4
  TorqueVectoringAlgorithm/1(NTorqueLeftOut) -> NTorqueLeftOut/1
  NTorqueMaxDeltaF/1 -> TorqueVectoringAlgorithm/2(NTorqueMaxDelta)
  vLat/1 -> Vehicle Slip Angle Error/1
  TorqueVectoringAlgorithm/2(NTorqueRightOut) -> NTorqueRightOut/1
  rRegenSplitF/1 -> TorqueSplit/2
  TorqueVectoringAlgorithm1/1(NTorqueLeftOut) -> NTorqueLeftOut1/1
  P_YR/1 -> TorqueVectoringAlgorithm1/6(P_YR), TorqueVectoringAlgorithm/6(P_YR)
  NTorqueMaxDeltaR/1 -> TorqueVectoringAlgorithm1/2(NTorqueMaxDelta)

== system TorqueVect/CarMaker/IPG Vehicle/PowerTrain/PTControl Example/PTControl_TV_MFE2/New TC ==
  lim 1 : Inport
  lim 2 : Inport  Port=2
  lim 3 : Inport  Port=3
  lim 4 : Inport  Port=4
  vx : Inport  Port=5
  w_FL : Inport  Port=6
  w_FR : Inport  Port=7
  w_RL : Inport  Port=8
  w_RR : Inport  Port=9
  Front SR Target : Inport  Port=10
  Rear SR Target : Inport  Port=11
  P_TC : Inport  Port=12
  D_TC : Inport  Port=13
  enable_tc : Inport  Port=14
  rate_h : Inport  Port=15
  rate_l : Inport  Port=16
  Demux1 : Demux
  Gain : Gain  Gain=0.2032/13.39
  Rate Limiter Dynamic{,1..3} (4 alike) : simulink/Discontinuities/Rate Limiter Dynamic
  Reference Generator1 : Subsystem
  Saturation : Saturate  UpperLimit=inf  LowerLimit=0
  Subtract1 : Sum  Inputs=-+
  TC R1 : Subsystem
  TC R2 : Subsystem
  TC R3 : Subsystem
  TC R4 : Subsystem
  Vector Concatenate3 : Concatenate  NumInputs=4
  R1 Demand : Outport
  L1 Demand : Outport  Port=2
  R2 Demand : Outport  Port=3
  L2 Demand : Outport  Port=4
  wires:
  Reference Generator1/1(R1) -> TC R1/1(modified slip ratio reference)
  lim 1/1 -> TC R1/2(lim 1)
  Gain/1 -> Subtract1/2
  Vector Concatenate3/1 -> Gain/1  "omega"
  Subtract1/1 -> Demux1/1
  vx/1 -> Saturation/1
  TC R2/1(Control Effort 1) -> Rate Limiter Dynamic1/2  "MMotorL1Demand"
  w_RL/1 -> Vector Concatenate3/4
  w_RR/1 -> Vector Concatenate3/3
  w_FL/1 -> Vector Concatenate3/2
  w_FR/1 -> Vector Concatenate3/1
  Front SR Target/1 -> Reference Generator1/2(Front SR Target)
  Rear SR Target/1 -> Reference Generator1/3(Rear SR Target)
  lim 2/1 -> TC R2/2(lim 1)
  lim 3/1 -> TC R3/2(lim 1)
  lim 4/1 -> TC R4/2(lim 1)
  Reference Generator1/2(L1) -> TC R2/1(modified slip ratio reference)
  Reference Generator1/3(R2) -> TC R3/1(modified slip ratio reference)
  Reference Generator1/4(L2) -> TC R4/1(modified slip ratio reference)
  P_TC/1 -> TC R2/4(P_TC), TC R4/4(P_TC), TC R3/4(P_TC), TC R1/4(P_TC)
  D_TC/1 -> TC R2/5(D_TC), TC R4/5(D_TC), TC R3/5(D_TC), TC R1/5(D_TC)
  Demux1/1 -> TC R1/3(modified slip ratio measurement)
  Demux1/2 -> TC R2/3(modified slip ratio measurement)
  Demux1/3 -> TC R3/3(modified slip ratio measurement)
  Demux1/4 -> TC R4/3(modified slip ratio measurement)
  TC R1/1(Control Effort 1) -> Rate Limiter Dynamic/2  "MMotorR1Demand"
  Saturation/1 -> Subtract1/1, Reference Generator1/1(x2)
  TC R3/1(Control Effort 1) -> Rate Limiter Dynamic2/2
  TC R4/1(Control Effort 1) -> Rate Limiter Dynamic3/2
  enable_tc/1 -> TC R4/6(enable_tc), TC R2/6(enable_tc), TC R3/6(enable_tc), TC R1/6(enable_tc)
  Rate Limiter Dynamic/1 -> R1 Demand/1
  rate_h/1 -> Rate Limiter Dynamic3/1, Rate Limiter Dynamic2/1, Rate Limiter Dynamic1/1, Rate Limiter Dynamic/1
  rate_l/1 -> Rate Limiter Dynamic/3, Rate Limiter Dynamic3/3, Rate Limiter Dynamic2/3, Rate Limiter Dynamic1/3
  Rate Limiter Dynamic1/1 -> L1 Demand/1
  Rate Limiter Dynamic2/1 -> R2 Demand/1
  Rate Limiter Dynamic3/1 -> L2 Demand/1

== system TorqueVect/CarMaker/IPG Vehicle/PowerTrain/PTControl Example/PTControl_TV_MFE2/PTC ==
  Constant2 : Constant
  Ground : Ground
  Mode_EngineDrive : Constant  Value=4
  Mux : Mux
  OperState_Driving : Constant  Value=4
  PTC MiscOut : Outport  VectorParamsAs1DForOutWhenUnconnected=off
  wires:
  Constant2/1 -> Mux/4  "Ignition"
  Mode_EngineDrive/1 -> Mux/3
  Ground/1 -> Mux/2  "OperationError"
  OperState_Driving/1 -> Mux/1
  Mux/1 -> PTC MiscOut/1

== system TorqueVect/CarMaker/IPG Vehicle/PowerTrain/PTControl Example/PTControl_TV_MFE2/Subsystem ==
  vLong : Inport
  aSteerWheel : Inport  Port=2
  vLongMin : Inport  Port=3
  aSteerWheelMin : Inport  Port=4
  NTorqueMaxDeltaF : Inport  Port=5
  BTorqueVectoringEnable : Inport  Port=6
  P_YR : Inport  Port=7
  D_YR : Inport  Port=8
  NBrake : Inport  Port=9
  rThrottle : Inport  Port=10
  MMotorMax : Inport  Port=11
  vLat : Inport  Port=12
  rSteerWheel : Inport  Port=13
  NTorqueMaxDeltaR : Inport  Port=14
  Add : Sum
  Add1 : Sum
  Constant : Constant  Value=-10
  Constant1 : Constant  Value=0.4
  PedalConversion : Subsystem
  Subsystem : Subsystem
  TV Enable Checker : Subsystem
  TorqueSplit : Subsystem
  TorqueVectoringAlgorithm : Subsystem  AncestorBlock=TorqueVectoringLibrary/TorqueVectoringAlgorithm
  TorqueVectoringAlgorithm1 : Subsystem  AncestorBlock=TorqueVectoringLibrary/TorqueVectoringAlgorithm
  NTorqueLeftOut : Outport
  NTorqueRightOut : Outport  Port=2
  NTorqueLeftOut1 : Outport  Port=3
  NTorqueRightOut1 : Outport  Port=4
  aSlip : Outport  Port=5
  wires:
  Subsystem/1(aSlip) -> aSlip/1, TorqueVectoringAlgorithm1/5(aSlip), TorqueVectoringAlgorithm/5(aSlip)
  TorqueSplit/3(MMotorDemandRL) -> Add1/2
  BTorqueVectoringEnable/1 -> TV Enable Checker/5(BTorqueVectoringEnable)
  TorqueSplit/2(MMotorDemandFR) -> Add/2
  TV Enable Checker/1(BEnable) -> TorqueVectoringAlgorithm1/1(BEnable), TorqueVectoringAlgorithm/1(BEnable)  "Enable"
  rSteerWheel/1 -> Subsystem/4(rSteerWheel)
  Add1/1 -> TorqueVectoringAlgorithm1/4(NTorqueAxle)
  TorqueVectoringAlgorithm1/2(NTorqueRightOut) -> NTorqueRightOut1/1
  NBrake/1 -> TorqueVectoringAlgorithm/8(NBrake), TorqueVectoringAlgorithm1/8(NBrake)
  Add/1 -> TorqueVectoringAlgorithm/4(NTorqueAxle)
  TorqueSplit/4(MMotorDemandRR) -> Add1/1
  vLong/1 -> Subsystem/2(vLong), TV Enable Checker/1(vLong)
  TorqueSplit/1(MMotorDemandFL) -> Add/1
  aSteerWheel/1 -> Subsystem/3(aSteerWheel), TV Enable Checker/2(aSteerWheel)
  vLongMin/1 -> TV Enable Checker/3(vLongMin)
  aSteerWheelMin/1 -> TV Enable Checker/4(aSteerWheelMin)
  D_YR/1 -> TorqueVectoringAlgorithm/7(D_YR), TorqueVectoringAlgorithm1/7(D_YR)
  MMotorMax/1 -> TorqueSplit/3(MMotorMax), TorqueVectoringAlgorithm/3(NTorqueMax), TorqueVectoringAlgorithm1/3(NTorqueMax)
  TorqueVectoringAlgorithm/1(NTorqueLeftOut) -> NTorqueLeftOut/1
  NTorqueMaxDeltaF/1 -> TorqueVectoringAlgorithm/2(NTorqueMaxDelta)
  vLat/1 -> Subsystem/1(vLat)
  TorqueVectoringAlgorithm/2(NTorqueRightOut) -> NTorqueRightOut/1
  TorqueVectoringAlgorithm1/1(NTorqueLeftOut) -> NTorqueLeftOut1/1
  P_YR/1 -> TorqueVectoringAlgorithm1/6(P_YR), TorqueVectoringAlgorithm/6(P_YR)
  NTorqueMaxDeltaR/1 -> TorqueVectoringAlgorithm1/2(NTorqueMaxDelta)
  Constant/1 -> TorqueSplit/4(MRegenMotorMax)
  rThrottle/1 -> PedalConversion/1(rThrottlePedal)
  PedalConversion/1(rThrottle) -> TorqueSplit/2(rThrottle)
  Constant1/1 -> TorqueSplit/1(rSplitF)

== system TorqueVect/CarMaker/IPG Vehicle/PowerTrain/PTControl Example/PTControl_TV_MFE25/Full Control Loop ==
  l_lim : Inport
  ResetSignal : Inport  Port=2
  u : Inport  Port=3
  Fz_per_wheel : Inport  Port=4
  vehicle_speed : Inport  Port=5
  min_speed : Inport  Port=6
  P_max : Inport  Port=7
  T_i_max : Inport  Port=8
  lamda : Inport  Port=9
  omega : Inport  Port=10
  efficiency : Inport  Port=11
  Demux : Demux
  MATLAB Function : MATLAB Function  TreatAsAtomicUnit=on
  Multiply : Gain  Gain=0.2
  Product : Product
  Reference Generator : Subsystem
  Subtract : Sum  Inputs=+-
  TC 1 : Subsystem
  TC 2 : Subsystem
  TC 3 : Subsystem
  TC 4 : Subsystem
  Torque Allocation : MATLAB Function  Commented=on  TreatAsAtomicUnit=on
  \tau_1 : Outport
  \tau_2 : Outport  Port=2
  \tau_3 : Outport  Port=3
  \tau_4 : Outport  Port=4
  wires:
  T_i_max/1 -> Torque Allocation/5(T_i_max), MATLAB Function/5(T_i_max)  "u4"
  u/1 -> MATLAB Function/2(u), Torque Allocation/2(u), Reference Generator/1(u)
  Reference Generator/2(r2) -> TC 2/1(modified slip ratio reference)  "r2"
  TC 2/1(Control Effort 1) -> \tau_2/1  "\\tau_2"
  TC 3/1(Control Effort 1) -> \tau_3/1  "\\tau_3"
  Fz_per_wheel/1 -> MATLAB Function/1(F), Torque Allocation/1(F), Reference Generator/2(Fz_per_wheel)
  lamda/1 -> Torque Allocation/6(lamda), MATLAB Function/6(lamda)
  vehicle_speed/1 -> Subtract/2, TC 2/6(velocity), TC 4/6(velocity), TC 3/6(velocity), TC 1/6(velocity), Reference Generator/3(vehicle_speed)
  P_max/1 -> Product/2
  l_lim/1 -> TC 2/4(l_lim), TC 4/4(l_lim), TC 3/4(l_lim), TC 1/4(l_lim)
  Reference Generator/3(r3) -> TC 3/1(modified slip ratio reference)  "r3"
  Subtract/1 -> Demux/1
  omega/1 -> MATLAB Function/3(omega), Torque Allocation/3(omega), Multiply/1
  Demux/4 -> TC 4/3(modified slip ratio measurement)  "msr4"
  TC 1/1(Control Effort 1) -> \tau_1/1  "\\tau_1"
  ResetSignal/1 -> TC 2/5(ResetSignal), TC 4/5(ResetSignal), TC 3/5(ResetSignal), TC 1/5(ResetSignal)
  Reference Generator/4(r4) -> TC 4/1(modified slip ratio reference)  "r4"
  min_speed/1 -> Reference Generator/4(min_speed)
  TC 4/1(Control Effort 1) -> \tau_4/1  "\\tau_4"
  Demux/3 -> TC 3/3(modified slip ratio measurement)  "msr3"
  Multiply/1 -> Subtract/1
  Demux/1 -> TC 1/3(modified slip ratio measurement)  "msr1"
  Demux/2 -> TC 2/3(modified slip ratio measurement)  "msr2"
  Reference Generator/1(r1) -> TC 1/1(modified slip ratio reference)  "r1"
  efficiency/1 -> Product/1
  Product/1 -> Torque Allocation/4(P_max), MATLAB Function/4(P_max)
  MATLAB Function/1(u1) -> TC 1/2(u_lim)  "y1"
  MATLAB Function/2(u2) -> TC 2/2(u_lim)  "y2"
  MATLAB Function/3(u3) -> TC 3/2(u_lim)  "y3"
  MATLAB Function/4(u4) -> TC 4/2(u_lim)  "y4"

== system TorqueVect/CarMaker/IPG Vehicle/PowerTrain/PTControl Example/PTControl_TV_MFE25/New TC ==
  lim 1 : Inport
  lim 2 : Inport  Port=2
  lim 3 : Inport  Port=3
  lim 4 : Inport  Port=4
  vx : Inport  Port=5
  w_FL : Inport  Port=6
  w_FR : Inport  Port=7
  w_RL : Inport  Port=8
  w_RR : Inport  Port=9
  Front SR Target : Inport  Port=10
  Rear SR Target : Inport  Port=11
  P_TC : Inport  Port=12
  D_TC : Inport  Port=13
  enable_tc : Inport  Port=14
  rate_h : Inport  Port=15
  rate_l : Inport  Port=16
  Demux1 : Demux
  Gain : Gain  Gain=0.2032/13.39
  Rate Limiter Dynamic{,1..3} (4 alike) : simulink/Discontinuities/Rate Limiter Dynamic
  Reference Generator1 : Subsystem
  Saturation : Saturate  UpperLimit=inf  LowerLimit=0
  Subtract1 : Sum  Inputs=-+
  TC R1 : Subsystem
  TC R2 : Subsystem
  TC R3 : Subsystem
  TC R4 : Subsystem
  Vector Concatenate3 : Concatenate  NumInputs=4
  R1 Demand : Outport
  L1 Demand : Outport  Port=2
  R2 Demand : Outport  Port=3
  L2 Demand : Outport  Port=4
  wires:
  Reference Generator1/1(R1) -> TC R1/1(modified slip ratio reference)
  lim 1/1 -> TC R1/2(lim 1)
  Gain/1 -> Subtract1/2
  Vector Concatenate3/1 -> Gain/1  "omega"
  Subtract1/1 -> Demux1/1
  vx/1 -> Saturation/1
  TC R2/1(Control Effort 1) -> Rate Limiter Dynamic1/2  "MMotorL1Demand"
  w_RL/1 -> Vector Concatenate3/4
  w_RR/1 -> Vector Concatenate3/3
  w_FL/1 -> Vector Concatenate3/2
  w_FR/1 -> Vector Concatenate3/1
  Front SR Target/1 -> Reference Generator1/2(Front SR Target)
  Rear SR Target/1 -> Reference Generator1/3(Rear SR Target)
  lim 2/1 -> TC R2/2(lim 1)
  lim 3/1 -> TC R3/2(lim 1)
  lim 4/1 -> TC R4/2(lim 1)
  Reference Generator1/2(L1) -> TC R2/1(modified slip ratio reference)
  Reference Generator1/3(R2) -> TC R3/1(modified slip ratio reference)
  Reference Generator1/4(L2) -> TC R4/1(modified slip ratio reference)
  P_TC/1 -> TC R2/4(P_TC), TC R4/4(P_TC), TC R3/4(P_TC), TC R1/4(P_TC)
  D_TC/1 -> TC R2/5(D_TC), TC R4/5(D_TC), TC R3/5(D_TC), TC R1/5(D_TC)
  Demux1/1 -> TC R1/3(modified slip ratio measurement)
  Demux1/2 -> TC R2/3(modified slip ratio measurement)
  Demux1/3 -> TC R3/3(modified slip ratio measurement)
  Demux1/4 -> TC R4/3(modified slip ratio measurement)
  TC R1/1(Control Effort 1) -> Rate Limiter Dynamic/2  "MMotorR1Demand"
  Saturation/1 -> Subtract1/1, Reference Generator1/1(x2)
  TC R3/1(Control Effort 1) -> Rate Limiter Dynamic2/2
  TC R4/1(Control Effort 1) -> Rate Limiter Dynamic3/2
  enable_tc/1 -> TC R4/6(enable_tc), TC R2/6(enable_tc), TC R3/6(enable_tc), TC R1/6(enable_tc)
  Rate Limiter Dynamic/1 -> R1 Demand/1
  rate_h/1 -> Rate Limiter Dynamic3/1, Rate Limiter Dynamic2/1, Rate Limiter Dynamic1/1, Rate Limiter Dynamic/1
  rate_l/1 -> Rate Limiter Dynamic/3, Rate Limiter Dynamic3/3, Rate Limiter Dynamic2/3, Rate Limiter Dynamic1/3
  Rate Limiter Dynamic1/1 -> L1 Demand/1
  Rate Limiter Dynamic2/1 -> R2 Demand/1
  Rate Limiter Dynamic3/1 -> L2 Demand/1

== system TorqueVect/CarMaker/IPG Vehicle/PowerTrain/PTControl Example/PTControl_TV_MFE25/PTC ==
  Constant2 : Constant
  Ground : Ground
  Mode_EngineDrive : Constant  Value=4
  Mux : Mux
  OperState_Driving : Constant  Value=4
  PTC MiscOut : Outport  VectorParamsAs1DForOutWhenUnconnected=off
  wires:
  Constant2/1 -> Mux/4  "Ignition"
  Mode_EngineDrive/1 -> Mux/3
  Ground/1 -> Mux/2  "OperationError"
  OperState_Driving/1 -> Mux/1
  Mux/1 -> PTC MiscOut/1

== system TorqueVect/CarMaker/IPG Vehicle/PowerTrain/PTControl Example/PTControl_TV_MFE25_2022a1/New TC ==
  lim 1 : Inport
  lim 2 : Inport  Port=2
  lim 3 : Inport  Port=3
  lim 4 : Inport  Port=4
  vx : Inport  Port=5
  w_FL : Inport  Port=6
  w_FR : Inport  Port=7
  w_RL : Inport  Port=8
  w_RR : Inport  Port=9
  Front SR Target : Inport  Port=10
  Rear SR Target : Inport  Port=11
  P_TC : Inport  Port=12
  D_TC : Inport  Port=13
  enable_tc : Inport  Port=14
  rate_h : Inport  Port=15
  rate_l : Inport  Port=16
  Demux1 : Demux
  Gain : Gain  Gain=0.2032/13.39
  Rate Limiter Dynamic{,1..3} (4 alike) : simulink/Discontinuities/Rate Limiter Dynamic
  Reference Generator1 : Subsystem
  Saturation : Saturate  UpperLimit=inf  LowerLimit=0
  Subtract1 : Sum  Inputs=-+
  TC R1 : Subsystem
  TC R2 : Subsystem
  TC R3 : Subsystem
  TC R4 : Subsystem
  Vector Concatenate3 : Concatenate  NumInputs=4
  R1 Demand : Outport
  L1 Demand : Outport  Port=2
  R2 Demand : Outport  Port=3
  L2 Demand : Outport  Port=4
  wires:
  Reference Generator1/1(R1) -> TC R1/1(modified slip ratio reference)
  lim 1/1 -> TC R1/2(lim 1)
  Gain/1 -> Subtract1/2
  Vector Concatenate3/1 -> Gain/1  "omega"
  Subtract1/1 -> Demux1/1
  vx/1 -> Saturation/1
  TC R2/1(Control Effort 1) -> Rate Limiter Dynamic1/2  "MMotorL1Demand"
  w_RL/1 -> Vector Concatenate3/4
  w_RR/1 -> Vector Concatenate3/3
  w_FL/1 -> Vector Concatenate3/2
  w_FR/1 -> Vector Concatenate3/1
  Front SR Target/1 -> Reference Generator1/2(Front SR Target)
  Rear SR Target/1 -> Reference Generator1/3(Rear SR Target)
  lim 2/1 -> TC R2/2(lim 1)
  lim 3/1 -> TC R3/2(lim 1)
  lim 4/1 -> TC R4/2(lim 1)
  Reference Generator1/2(L1) -> TC R2/1(modified slip ratio reference)
  Reference Generator1/3(R2) -> TC R3/1(modified slip ratio reference)
  Reference Generator1/4(L2) -> TC R4/1(modified slip ratio reference)
  P_TC/1 -> TC R2/4(P_TC), TC R4/4(P_TC), TC R3/4(P_TC), TC R1/4(P_TC)
  D_TC/1 -> TC R2/5(D_TC), TC R4/5(D_TC), TC R3/5(D_TC), TC R1/5(D_TC)
  Demux1/1 -> TC R1/3(modified slip ratio measurement)
  Demux1/2 -> TC R2/3(modified slip ratio measurement)
  Demux1/3 -> TC R3/3(modified slip ratio measurement)
  Demux1/4 -> TC R4/3(modified slip ratio measurement)
  TC R1/1(Control Effort 1) -> Rate Limiter Dynamic/2  "MMotorR1Demand"
  Saturation/1 -> Subtract1/1, Reference Generator1/1(x2)
  TC R3/1(Control Effort 1) -> Rate Limiter Dynamic2/2
  TC R4/1(Control Effort 1) -> Rate Limiter Dynamic3/2
  enable_tc/1 -> TC R4/6(enable_tc), TC R2/6(enable_tc), TC R3/6(enable_tc), TC R1/6(enable_tc)
  Rate Limiter Dynamic/1 -> R1 Demand/1
  rate_h/1 -> Rate Limiter Dynamic3/1, Rate Limiter Dynamic2/1, Rate Limiter Dynamic1/1, Rate Limiter Dynamic/1
  rate_l/1 -> Rate Limiter Dynamic/3, Rate Limiter Dynamic3/3, Rate Limiter Dynamic2/3, Rate Limiter Dynamic1/3
  Rate Limiter Dynamic1/1 -> L1 Demand/1
  Rate Limiter Dynamic2/1 -> R2 Demand/1
  Rate Limiter Dynamic3/1 -> L2 Demand/1

== system TorqueVect/CarMaker/IPG Vehicle/PowerTrain/PTControl Example/PTControl_TV_MFE25_2022a1/PTC ==
  Constant2 : Constant
  Ground : Ground
  Mode_EngineDrive : Constant  Value=4
  Mux : Mux
  OperState_Driving : Constant  Value=4
  PTC MiscOut : Outport  VectorParamsAs1DForOutWhenUnconnected=off
  wires:
  Constant2/1 -> Mux/4  "Ignition"
  Mode_EngineDrive/1 -> Mux/3
  Ground/1 -> Mux/2  "OperationError"
  OperState_Driving/1 -> Mux/1
  Mux/1 -> PTC MiscOut/1
